simulink model "EKF_MODEL_needfix"  (R2023b)
settings: Solver=ode23tb  StartTime=0.0  StopTime=30  FixedStep=.001  RelTol=2e-1  EnableMultiTasking=on
StartFcn:
  | %tic
StopFcn:
  | %toc
model workspace (MAT data in the model file):
  DLCXref = [0 6.1 6.2 18 33 33.5 45 50 60]
  DLCXrefStanley = [0 1.2 2.4 3.6 4.8 6 7.2 8.4 9.44987166868 10.0991210544 10.1 10.1008789456 ... (38 elements, 1x38)]
  DLCYref = [0 0 -5 -3.875 -3.5 1 0 0 0]
  DLCYrefStanley = [0.1375 0.1375 0.1375 0.1375 0.1375 0.1375 0.1375 0.1375 -0.203439148031 -1.09615705337 -2.2 -3.30384294663 ... (38 elements, 1x38)]
  Downshift_Speeds = [9.5625 12.9375 16.3125 19.6875 23.0625 26.4375 29.8125 33.1875 36.5625 39.9375 43.3125 46.6875 ... (28 elements, 4x7)]
  EngRevLim = 7000
  Pedal_Positions = [0.1 0.4 0.5 0.9]
  Ts = 0.01
  Upshift_Speeds = [12.9375 16.3125 19.6875 33 26.4375 29.8125 33.1875 52.5 39.9375 43.3125 46.6875 77.25 ... (28 elements, 4x7)]
  VEH : object (value not decoded)
  a = 1.515
  b = 1.504
  for_ekf : mamfis (value not decoded)
  rayDirections = [0 0 0 0 0 0 0 0 0 0 0 0 ... (363 elements, 121x3)]
  rayLengths = [20 20 20 20 20 20 20 20 20 20 20 20 ... (121 elements, 121x1)]
  rayOrigins = [0.5 0.4 0.3 0.2 0.1 0 -0.1 -0.2 -0.3 -0.4 -0.5 0.5 ... (363 elements, 121x3)]
  theta = 1
  wf = 0.75
  wr = 1.25
symbols that are objects in the model workspace (value not decoded): VEH
undefined symbols (not defined in the file): DiscIntNeverNeededParam
libraries: simulink x14, autolibutils x7, slpidlib x2, vehdynlibdriver x2, vehdynlibviscommon x2, sim3dgroundtruthsensorlib x2, autolibtranscontrolscommon x1, autolibshared x1, sharedtransform x1, sharedTrackingLibrary x1, vehdynlibscenariocommon x1, vehdynlibsens x1
(part 3 of 4)

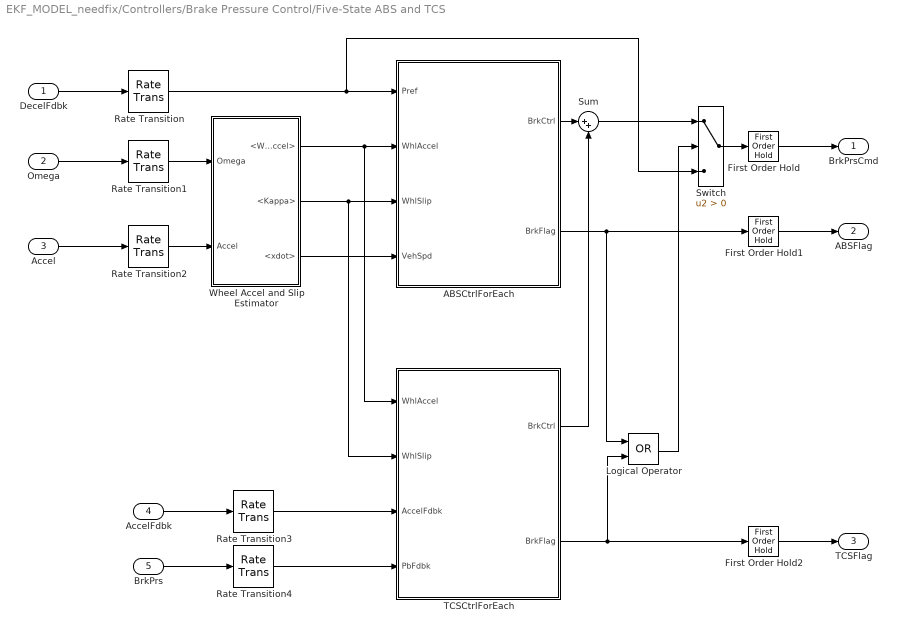
== system EKF_MODEL_needfix/Controllers/Brake Pressure Control/Five-State ABS and TCS ==
  DecelFdbk : Inport
  Omega : Inport  Port=2
  Accel : Inport  Port=3
  AccelFdbk : Inport  Port=4
  BrkPrs : Inport  Port=5
  ABSCtrlForEach : Subsystem  mask(Five-State ABS Control){Re=0.323, KappaOpt=-0.12, WhlAccelOpt=[-9.8,-9.8,-20,-20], v1=0, v5=0.55, v4=1, a2=-1.5, b=-1.5, A=4.5, a1=3.6, aMode=2}
      mask prompts: Re "Wheel effective radius, Re [m]:"; KappaOpt "Desired wheel slip ratio, KappaOpt [-]:"; WhlAccelOpt "Desired wheel acceleration, WhlAccelOpt [m/s^2]:"; v1 "Braking realease command, v1 [-]:"; v5 "Braking hold command, v5 [-]:"; v4 "Braking add command, v4 [-]:"; a2 "Threshold of State 1, a2 [m/s^2]:"; b "Threshold of State 2, b [m/s^2]:"; A "Threshold of State 3 and 4, A [m/s^2]:"; a1 "Threshold of State 5, a1 [m/s^2]:"
      mask help: This block determines brake pressure varying rate for each wheel once the ABS controller is activated. During ABS control, only wheel speed is directly regulated.
      mask init:
      | [~]=vehdynicon('vehdynblk',gcb);
      mask DialogControl vehParamGroup Prompt: Vehicle Parameter
      mask DialogControl ParameterGroupVar Prompt: Desired Control Parameters
      mask DialogControl Container3 Prompt: Braking Pressure Rates
      mask DialogControl Container4 Prompt: Wheel Acceleration Thresholds
  First Order Hold : FirstOrderHold  ErrorTolerance=.01
  First Order Hold1 : FirstOrderHold  ErrorTolerance=1
  First Order Hold2 : FirstOrderHold  ErrorTolerance=1
  Logical Operator : Logic  Operator=OR  AllPortsSameDT=off  OutDataTypeStr=boolean
  Rate Transition{,1..4} (5 alike) : RateTransition  OutPortSampleTime=.001
  Sum : Sum  Inputs=|++
  Switch : Switch  Criteria=u2 > Threshold  SaturateOnIntegerOverflow=off  InputSameDT=off
  TCSCtrlForEach : Subsystem  mask(Five-State TCS Control){Re=0.323, KappaOpt=0.12, WhlAccelOpt=[11, 11, 11, 11], v1=1.5, v5=-0.5, v4=-1.2, a2=-6, b=-10, A=-11, a1=-9, aMode=2}
      mask prompts: Re "Wheel effective radius, Re [m]:"; KappaOpt "Desired wheel slip ratio, KappaOpt [-]:"; WhlAccelOpt "Desired wheel acceleration, WhlAccelOpt [m/s^2]:"; v1 "Braking pressure rising rate, v1 [-]:"; v5 "Secondary braking pressure declining rate, v5 [-]:"; v4 "Braking pressure declining rate, v4 [-]:"; a2 "Threshold of State 1, a2 [m/s^2]:"; b "Threshold of State 2, b [m/s^2]:"; A "Threshold of State 3 and 4, A [m/s^2]:"; a1 "Threshold of State 5, a1 [m/s^2]:"
      mask help: This block determines brake pressure varying rate for each wheel once the TCS controller is activated. During TCS control, only wheel speed is directly regulated.
      mask init:
      | [~]=vehdynicon('vehdynblk',gcb);
      mask DialogControl vehParamGroup Prompt: Vehicle Parameter
      mask DialogControl ParameterGroupVar Prompt: Desired Control Parameters
      mask DialogControl Container3 Prompt: Braking Pressure Rates
      mask DialogControl Container4 Prompt: Wheel Acceleration Thresholds
  Wheel Accel and Slip Estimator : Subsystem
  BrkPrsCmd : Outport
  ABSFlag : Outport  Port=2  PortDimensions=4
  TCSFlag : Outport  Port=3  PortDimensions=4
  wires:
  Omega/1 -> Rate Transition1/1
  Accel/1 -> Rate Transition2/1
  DecelFdbk/1 -> Rate Transition/1
  Wheel Accel and Slip Estimator/1(<WhlAccel>) -> TCSCtrlForEach/1(WhlAccel), ABSCtrlForEach/2(WhlAccel)
  Wheel Accel and Slip Estimator/2(<Kappa>) -> TCSCtrlForEach/2(WhlSlip), ABSCtrlForEach/3(WhlSlip)
  Wheel Accel and Slip Estimator/3(<xdot>) -> ABSCtrlForEach/4(VehSpd)
  ABSCtrlForEach/2(BrkFlag) -> First Order Hold1/1, Logical Operator/1
  First Order Hold/1 -> BrkPrsCmd/1
  Rate Transition/1 -> Switch/3, ABSCtrlForEach/1(Pref)
  Rate Transition1/1 -> Wheel Accel and Slip Estimator/1(Omega)
  Rate Transition2/1 -> Wheel Accel and Slip Estimator/2(Accel)
  First Order Hold1/1 -> ABSFlag/1
  Switch/1 -> First Order Hold/1
  AccelFdbk/1 -> Rate Transition3/1
  First Order Hold2/1 -> TCSFlag/1
  TCSCtrlForEach/2(BrkFlag) -> First Order Hold2/1, Logical Operator/2
  Rate Transition3/1 -> TCSCtrlForEach/3(AccelFdbk)
  TCSCtrlForEach/1(BrkCtrl) -> Sum/2
  ABSCtrlForEach/1(BrkCtrl) -> Sum/1
  BrkPrs/1 -> Rate Transition4/1
  Rate Transition4/1 -> TCSCtrlForEach/4(PbFdbk)
  Sum/1 -> Switch/1
  Logical Operator/1 -> Switch/2

== system EKF_MODEL_needfix/Controllers/Brake Pressure Control/Open Loop ==
  DecelFdbk : Inport
  Constant : Constant  Value=false
  Selector : Selector  InputPortWidth=1  IndexOptions=Index vector (dialog)  Indices=[1 1 1 1]  OutputSizes=1
  Selector1 : Selector  InputPortWidth=1  IndexOptions=Index vector (dialog)  Indices=[1 1 1 1]  OutputSizes=1
  BrkPrsCmd : Outport  VectorParamsAs1DForOutWhenUnconnected=off
  ABSFlag : Outport  Port=2
  wires:
  DecelFdbk/1 -> Selector1/1
  Selector1/1 -> BrkPrsCmd/1
  Constant/1 -> Selector/1
  Selector/1 -> ABSFlag/1

== system EKF_MODEL_needfix/Controllers/ECU/Torque Cmd ==
  DiffTrqCmd : Inport
  <Accel> : Inport  Port=2
  EngSpd : Inport  Port=3
  ABSFlag : Inport  Port=4
  Acc to Torque Request : Gain  Gain=150
  Constant : Constant  Value=0
  Max : MinMax  Function=max  Inputs=2
  OR : Logic  Operator=OR  Inputs=1  AllPortsSameDT=off  OutDataTypeStr=boolean
  Rev Limiter Control : Subsystem
  Signal Specification : SignalSpecification  Unit=rpm
  Switch : Switch  Criteria=u2 > Threshold  ZeroCross=off  SaturateOnIntegerOverflow=off  InputSameDT=off
  Unit Conversion : UnitConversion
  EngTrqCmd : Outport
  wires:
  Signal Specification/1 -> Rev Limiter Control/2(EngSpd)  "EngSpd"
  Unit Conversion/1 -> Signal Specification/1
  EngSpd/1 -> Unit Conversion/1
  <Accel>/1 -> Acc to Torque Request/1
  Acc to Torque Request/1 -> Rev Limiter Control/1(TrqCmd)
  DiffTrqCmd/1 -> Max/1
  Rev Limiter Control/1(TrqCmdRevLimited) -> Max/2
  Switch/1 -> EngTrqCmd/1
  Max/1 -> Switch/3
  ABSFlag/1 -> OR/1
  Constant/1 -> Switch/1
  OR/1 -> Switch/2

== system EKF_MODEL_needfix/Controllers/Transmission Controller/Driver - No Clutch ==
  GearReq : Inport
  Gear : Outport  VectorParamsAs1DForOutWhenUnconnected=off
  wires:
  GearReq/1 -> Gear/1

== system EKF_MODEL_needfix/Controllers/Transmission Controller/PRNDL Controller ==
  Accel : Inport
  BrkCmd : Inport  Port=2
  Omega : Inport  Port=3  Unit=rad/s
  EngSpd : Inport  Port=4  Unit=rad/s
  GearReq : Inport  Port=5
  ABSFlag : Inport  Port=6
  Cont LPF : autolibutils/Cont LPF  wc=4*2*pi  AbsoluteTolerance=auto  aMode=2
  Cont LPF1 : autolibutils/Cont LPF  wc=4*2*pi  AbsoluteTolerance=auto  aMode=2
  Gain : Gain  Gain=.3065/4
  OR : Logic  Operator=OR  Inputs=1  AllPortsSameDT=off  OutDataTypeStr=boolean
  Signal Specification1 : SignalSpecification  Unit=m/s
  Sum of Elements : Sum  Inputs=+
  Transmission Controller PRNDL : autolibtranscontrolscommon/Transmission Controller PRNDL  DriveMode=off  GearInit=1  LugSpd=1200  MinUpSpd=2000  tClutchUp=0.5  tClutchDn=0.5  tPark=120  VelUnit=km/hr  UpShSpd="reshape([20    25    30    45    35    45    40    55    40    55    55    65    50    60    65    75    60    65    80    90    70    75   120   150    85    85   150   185  20    25    30    45    35    45    40    55    40    55    55    65    50    60    65    75    60    65    80    90    70    75   120   150    85    85   150   185],4,7,2)"  UpLdBpt=[.1 .4 .75 1]  UpShBpt=1:7  UpPtBpt=[1 2]  DnShfSpd=reshape([9.5625 12.9375 16.3125 19.6875 23.0625 26.4375 29.8125 33.1875 36.5625 39.9375 43.3125 46.687499999999986 47.8125 51.187499999999986 54.562499999999986 57.9375 59.0625 62.4375 65.8125 69.1875 68.90625 72.84375 76.78125 80.71875 78.75 83.25 87.75 92.25 31.619930749150555 36.119930749150555 37.619930749150555 43.619930749150555 44.318578948924035 48.818578948924035 50.318578948924035 56.318578948924035 53.598360325681568 58.098360325681568 59.598360325681568 65.598360325681568 66.252607657623685 70.752607657623685 72.252607657623685 78.252607657623685 84.53096491487338 89.03096491487338 90.53096491487338 96.53096491487338 134.79644737231007 139.29644737231007 140.79644737231007 146.79644737231007 210.1946710584651 214.6946710584651 216.1946710584651 222.1946710584651],4,7,2)  DnShSpd=[10 15 25 30 40 55 75; 10 18 25 35 50 65 80; 12 18 21 55 65 75 85; 15 20 25 55 70 80 95]  DnLdBpt=[.1 .4 .75 1]  DnShBpt=2:8  DnPtBpt=[1 2]  POFS=zeros(4,1)  GOFS=zeros(1,7)  Ngears=8  aMode=2
  Gear : Outport  VectorParamsAs1DForOutWhenUnconnected=off
  wires:
  Gain/1 -> Cont LPF1/1
  Omega/1 -> Sum of Elements/1
  Sum of Elements/1 -> Gain/1
  ABSFlag/1 -> OR/1
  OR/1 -> Transmission Controller PRNDL/6
  Transmission Controller PRNDL/1 -> Gear/1
  GearReq/1 -> Transmission Controller PRNDL/1  "PRNDL"
  Accel/1 -> Transmission Controller PRNDL/2
  BrkCmd/1 -> Transmission Controller PRNDL/3
  Signal Specification1/1 -> Transmission Controller PRNDL/4
  EngSpd/1 -> Cont LPF/1
  Cont LPF1/1 -> Signal Specification1/1
  Cont LPF/1 -> Transmission Controller PRNDL/5

== system EKF_MODEL_needfix/Controllers/Transmission Controller/Paddles ==
  Accel : Inport
  EngSpd : Inport  Port=2  Unit=rad/s
  Add1 : Sum  Inputs=+-+
  Current Gear : UnitDelay  SampleTime=-1  HasFrameUpgradeWarning=on
  Data Type Conversion2 : DataTypeConversion  OutDataTypeStr=double  SaturateOnIntegerOverflow=off  RndMeth=Floor
  Debounce : autolibutils/Debounce  DbcOn_Cnts=10  DbcOff_Cnts=10  aMode=aMode
  Debounce1 : autolibutils/Debounce  DbcOn_Cnts=10  DbcOff_Cnts=10  aMode=aMode
  Demux : Demux  Outputs=2
  Detect Increase2 : simulink/Logic and Bit Operations/Detect Increase  vinit=0.0  OutDataTypeStr=boolean
  Logical Operator1 : Logic  Operator=XOR  Inputs=1  AllPortsSameDT=off  OutDataTypeStr=boolean
  Mux : Mux  Inputs=2
  Switch2 : Switch  Criteria=u2 > Threshold  SaturateOnIntegerOverflow=off  InputSameDT=off
  Gear : Outport  VectorParamsAs1DForOutWhenUnconnected=off
  wires:
  Debounce/1 -> Mux/1
  Mux/1 -> Detect Increase2/1
  Logical Operator1/1 -> Switch2/2
  Data Type Conversion2/1 -> Demux/1
  Demux/1 -> Add1/1
  Demux/2 -> Add1/2
  Current Gear/1 -> Add1/3, Switch2/3
  Switch2/1 -> Gear/1, Current Gear/1
  Debounce1/1 -> Mux/2
  Add1/1 -> Switch2/1
  Detect Increase2/1 -> Data Type Conversion2/1, Logical Operator1/1
  EngSpd/1 -> Debounce1/1
  Accel/1 -> Debounce/1

== system EKF_MODEL_needfix/Controllers/Transmission Controller/Transmission Controller ==
  Accel : Inport
  EngSpd : Inport  Port=2  Unit=rad/s
  Omega : Inport  Port=3  Unit=rad/s
  10ms Function-Call Generator : simulink/Ports & Subsystems/Function-Call Generator  sample_time=0.01  numberOfIterations=1  DisallowWideOutput=off
  Data Type Conversion : DataTypeConversion  SaturateOnIntegerOverflow=off  RndMeth=Floor
  First Order Hold : FirstOrderHold  ErrorTolerance=.1
  Rate Transition : RateTransition  Deterministic=off
  Rate Transition1 : RateTransition  Deterministic=off
  Rate Transition2 : RateTransition  Deterministic=off
  Signal Specification : SignalSpecification  Unit=rpm
  TCM : Subsystem
  Unit Conversion : UnitConversion
  Gear : Outport  VectorParamsAs1DForOutWhenUnconnected=off
  wires:
  TCM/1(GearCmd) -> Data Type Conversion/1
  Rate Transition/1 -> TCM/1(AccCmd)
  10ms Function-Call Generator/1 -> TCM/Trigger
  Accel/1 -> Rate Transition/1
  Omega/1 -> Rate Transition2/1
  Rate Transition1/1 -> TCM/2(EngSpd)
  First Order Hold/1 -> Gear/1
  Unit Conversion/1 -> Signal Specification/1
  Signal Specification/1 -> Rate Transition1/1  "EngSpd"
  EngSpd/1 -> Unit Conversion/1
  Data Type Conversion/1 -> First Order Hold/1
  Rate Transition2/1 -> TCM/3(Omega)

== system EKF_MODEL_needfix/Driver Commands/Driver Commands/Longitudinal Driver ==
  VehRef : Inport
  VehFdbk : Inport  Port=2
  Bus Creator2 : BusCreator  Inputs=5
  Bus Selector2 : BusSelector  OutputSignals=Body.BdyFrm.Cg.Vel.xdot,Body.InertFrm.Cg.Disp.X
  Bus Selector3 : BusSelector  OutputSignals=SteerOvrCmd,LngRef,LtrlRef
  Dead Zone1 : DeadZone  LowerValue=-.1  UpperValue=.1
  Ground1 : Ground
  Ground2 : Ground
  Longitudinal Driver : autolibshared/Longitudinal Driver  extAccelOvr=off  extDecelOvr=off  extAccelHld=off  extDecelHld=off  extAccelZero=off  extDecelZero=off  cntrlType=Predictive  shftType=Reverse, Neutral, Drive  velUnits=m/s  gearOut=on  Kp=5  Ki=5  Kff=.1  Kg=0  VehVelVec=[0 100]  KffVec=[.1 .1]  KpVec=[10 10]  KiVec=[5 5]  KgVec=[0 0]  m=VEH.Mass  Kpt=3000  tau=.5  L=2  aR=200  bR=2.5  cR=.5  g=9.81  vnom=5  Kaw=1  tauerr=.1  tauPt=2  GearInit=0  tShift=.1  pdlVec=[0.1 0.4 0.5 0.9]  upShftTbl=[-1 12.9375 26.4375 39.9375 51.18749999999999 62.4375 72.84375 83.25;-1 16.3125 29.8125 43.3125 54.5624 65.8125 76.78125 87.75;-1 19.6875 33.1875 46.68749999999999 57.9375 69.1875 80.71875 92.25;-1 33 52.5 77.25 100.5 138.75 161.875 185]  dwnShftTbl=[1 9.5625 23.0625 36.5625 47.8125 59.0625 68.90625 78.75;1 12.9375 26.4375 39.9375 51.18749999999999 62.4375 72.84375 83.25;1 16.3125 29.8125 43.3125 54.562499 65.8125 76.78125 87.75;1 19.6875 33.1875 46.68749999999999 57.9375 69.1875 80.71875 92.25]  tClutch=.5  tRev=.5  tPark=120  aMode=2  UpGearVec="[0  1  2  3  4  5  6  7]"  DownGearVec="[1  2  3  4  5  6  7  8]"
      settings: LibrarySourceBlock=vehdynlibdriver/Longitudinal Driver
  Mux : Mux  Inputs=3
  Signal Copy : SignalConversion  OverrideOpt=off
  Terminator1 : Terminator
  Unit Conversion : UnitConversion
  Driver : Outport  VectorParamsAs1DForOutWhenUnconnected=off
  wires:
  VehRef/1 -> Bus Selector3/1
  Signal Copy/1 -> Bus Creator2/1  "SteerCmd"
  Longitudinal Driver/2 -> Bus Creator2/2  "AccelCmd"
  Dead Zone1/1 -> Longitudinal Driver/2
  Bus Selector3/2 -> Unit Conversion/1  "<LngRef>"
  Ground1/1 -> Longitudinal Driver/3
  Bus Selector2/1 -> Dead Zone1/1  "<xdot>"
  Bus Creator2/1 -> Driver/1
  Longitudinal Driver/1 -> Terminator1/1
  Longitudinal Driver/3 -> Bus Creator2/3  "DecelCmd"
  VehFdbk/1 -> Bus Selector2/1
  Bus Selector3/1 -> Signal Copy/1  "<SteerOvrCmd>"
  Ground2/1 -> Mux/3
  Bus Selector2/2 -> Mux/1  "<X>"
  Mux/1 -> Bus Creator2/5  "Ref"
  Bus Selector3/3 -> Mux/2  "<LtrlRef>"
  Longitudinal Driver/4 -> Bus Creator2/4  "GearCmd"
  Unit Conversion/1 -> Longitudinal Driver/1

== system EKF_MODEL_needfix/Driver Commands/Driver Commands/Open Loop ==
  VehFdbk : Inport
  SteerCmd : Inport  Port=2
  Accel : Inport  Port=3  Unit=one
  Brake : Inport  Port=4  Unit=1
  Gear : Inport  Port=5  Unit=1
  Bus Creator1 : BusCreator  Inputs=4
  Signal Specification : SignalSpecification  Unit=rad
  Signal Specification1 : SignalSpecification  Unit=1
  Signal Specification2 : SignalSpecification  Unit=1
  Signal Specification3 : SignalSpecification  Unit=1
  Terminator : Terminator
  Unit Conversion{,1..3} (4 alike) : UnitConversion
  Driver : Outport  VectorParamsAs1DForOutWhenUnconnected=off
  wires:
  Unit Conversion3/1 -> Signal Specification3/1
  Unit Conversion2/1 -> Signal Specification2/1
  Unit Conversion/1 -> Signal Specification/1
  Bus Creator1/1 -> Driver/1
  Accel/1 -> Unit Conversion1/1
  VehFdbk/1 -> Terminator/1
  SteerCmd/1 -> Unit Conversion/1
  Unit Conversion1/1 -> Signal Specification1/1
  Brake/1 -> Unit Conversion2/1
  Gear/1 -> Unit Conversion3/1
  Signal Specification/1 -> Bus Creator1/1  "SteerCmd"
  Signal Specification1/1 -> Bus Creator1/2  "AccelCmd"
  Signal Specification2/1 -> Bus Creator1/3  "DecelCmd"
  Signal Specification3/1 -> Bus Creator1/4  "GearCmd"

== system EKF_MODEL_needfix/Driver Commands/Driver Commands/Predictive Driver ==
  VehRef : Inport
  VehFdbk : Inport  Port=2
  Bus Creator1 : BusCreator  Inputs=5
  Bus Selector : BusSelector  OutputSignals=Body.BdyFrm.Cg.Vel.xdot,Body.InertFrm.Cg.Disp.Y,Body.BdyFrm.Cg.Vel.ydot,Body.InertFrm.Cg.Ang.psi,Body.BdyFrm.Cg.AngVel.r,Body.InertFrm.Cg.Disp.X
  Bus Selector1 : BusSelector  OutputSignals=LngRef,LtrlRef,EnblSteerCmd,SteerOvrCmd,AccelZero
  Dead Zone : DeadZone  LowerValue=-.5  UpperValue=.5  ZeroCross=off
  Grade : Constant  Value=0  SampleTime=-1
  Linear Predictive Driver : vehdynlibdriver/Predictive Driver  extAccelOvr=off  extDecelOvr=off  extAccelHld=off  extDecelHld=off  extAccelZero=on  extDecelZero=off  extSteerOvr=on  extSteerHld=off  extSteerZero=off  cntrlType=Predictive  cntrlTypeLat=Predictive  shftType=Reverse, Neutral, Drive  coordMode=SAE J670 (Z-down)  refType=Reference pose  velUnits=m/s  angUnits=rad  gearOut=on  steerOut=on  Kp=3  Ki=1  Kff=1  Kg=0  VehVelVec=[0 100]  KffVec=[.1 .1]  KpVec=[10 10]  KiVec=[5 5]  KgVec=[0 0]  vnom=5  Kaw=1  tauerr=.075  tau=.15  L=6  Kpt=20000  aR=200  bR=2.5  cR=.5  g=9.81  vecPose=off  dynamMode=on  PositionGainF=2.5  PositionGainR=2.5  YawRateGain=.2  DelayGain=.2  enableDrift=off  BetaRef=20*pi/180  KpBeta=1  KpDrift=2  KdDrift=1  KpPsi=6  KOmega=30  tOmega=1  a=VEH.FrontAxlePositionfromCG  b=VEH.RearAxlePositionfromCG  m=VEH.Mass  Cy_f=5000  Cy_r=7000  I=VEH.YawMomentInertia  Ksteer=18  theta=60*pi/180  Idl=1  Re=.3  lambda_mu=1  GearInit=0  tShift=.1  pdlVec=[0.1 0.4 0.5 0.9]  upShftTbl=[-1 12.9375 26.4375 39.9375 51.18749999999999 62.4375 72.84375 83.25;-1 16.3125 29.8125 43.3125 54.5624 65.8125 76.78125 87.75;-1 19.6875 33.1875 46.68749999999999 57.9375 69.1875 80.71875 92.25;-1 33 52.5 77.25 100.5 138.75 161.875 185]  dwnShftTbl=[-1 12.9375 26.4375 39.9375 51.18749999999999 62.4375 72.84375 83.25;-1 16.3125 29.8125 43.3125 54.5624 65.8125 76.78125 87.75;-1 19.6875 33.1875 46.68749999999999 57.9375 69.1875 80.71875 92.25;-1 33 52.5 77.25 100.5 138.75 161.875 185]  tClutch=.5  tRev=.5  tPark=120  UpGearVec="[0  1  2  3  4  5  6  7]"  DownGearVec="[1  2  3  4  5  6  7  8]"  aMode=2
  Mux : Mux  Inputs=3
  Terminator : Terminator
  Unit Conversion : UnitConversion
  Z : Constant  Value=0  SampleTime=-1
  Driver : Outport  VectorParamsAs1DForOutWhenUnconnected=off
  wires:
  Mux/1 -> Bus Creator1/5  "Ref"
  Bus Selector/6 -> Mux/1  "<X>"
  Linear Predictive Driver/5 -> Bus Creator1/4  "GearCmd"
  Bus Selector/3 -> Linear Predictive Driver/9  "<ydot>"
  Linear Predictive Driver/1 -> Terminator/1
  Bus Selector/5 -> Linear Predictive Driver/11  "<r>"
  Bus Selector1/2 -> Mux/2, Linear Predictive Driver/2  "<LtrlRef>"
  Z/1 -> Mux/3
  Grade/1 -> Linear Predictive Driver/6
  Bus Selector/1 -> Dead Zone/1  "<xdot>"
  Bus Selector/4 -> Linear Predictive Driver/10  "<psi>"
  Linear Predictive Driver/4 -> Bus Creator1/3  "DecelCmd"
  Dead Zone/1 -> Linear Predictive Driver/7
  VehFdbk/1 -> Bus Selector/1
  VehRef/1 -> Bus Selector1/1  "xdotref"
  Linear Predictive Driver/2 -> Bus Creator1/1  "SteerCmd"
  Bus Creator1/1 -> Driver/1
  Linear Predictive Driver/3 -> Bus Creator1/2  "AccelCmd"
  Bus Selector/2 -> Linear Predictive Driver/8  "<Y>"
  Bus Selector1/1 -> Unit Conversion/1  "<LngRef>"
  Bus Selector1/5 -> Linear Predictive Driver/5  "<AccelZero>"
  Bus Selector1/3 -> Linear Predictive Driver/3  "<EnblSteerCmd>"
  Bus Selector1/4 -> Linear Predictive Driver/4  "<SteerOvrCmd>"
  Unit Conversion/1 -> Linear Predictive Driver/1

== system EKF_MODEL_needfix/Driver Commands/Driver Commands/Predictive Stanley Driver ==
  VehRef : Inport
  VehFdbk : Inport  Port=2
  Bus Creator1 : BusCreator  Inputs=6
  Bus Selector : BusSelector  OutputSignals=Body.BdyFrm.Cg.Vel.xdot,Body.InertFrm.Cg.Disp.X,Body.InertFrm.Cg.Disp.Y,Body.InertFrm.Cg.Ang.psi,Body.BdyFrm.Cg.AngVel.r
  Bus Selector1 : BusSelector  OutputSignals=LngRef,PoseRef,EnblSteerCmd,SteerOvrCmd,SteerHld,SteerZero,EnblAccelOvr,AccelOvrCmd,AccelHld,AccelZero,EnblDecelCmd,DecelOvrCmd,DecelHld,DecelZero,CurvRef
  Constant : Constant  Value=false  SampleTime=-1
  Dead Zone : DeadZone  LowerValue=-.5  UpperValue=.5  ZeroCross=off
  Grade : Constant  Value=0  SampleTime=-1
  Linear Predictive Driver : vehdynlibdriver/Predictive Driver  extAccelOvr=on  extDecelOvr=on  extAccelHld=on  extDecelHld=on  extAccelZero=on  extDecelZero=on  extSteerOvr=on  extSteerHld=on  extSteerZero=on  cntrlType=Predictive  cntrlTypeLat=Stanley  shftType=Reverse, Neutral, Drive  coordMode=SAE J670 (Z-down)  refType=Reference pose  velUnits=m/s  angUnits=rad  gearOut=on  steerOut=on  Kp=3  Ki=1  Kff=1  Kg=0  VehVelVec=[0 100]  KffVec=[.1 .1]  KpVec=[10 10]  KiVec=[5 5]  KgVec=[0 0]  vnom=5  Kaw=1  tauerr=.075  tau=.15  L=6  Kpt=20000  aR=200  bR=2.5  cR=.5  g=9.81  vecPose=on  dynamMode=on  PositionGainF=2  PositionGainR=2  YawRateGain=.2  DelayGain=.01  enableDrift=off  BetaRef=20*pi/180  KpBeta=1  KpDrift=2  KdDrift=1  KpPsi=6  KOmega=30  tOmega=1  a=VEH.FrontAxlePositionfromCG  b=VEH.RearAxlePositionfromCG  m=VEH.Mass  Cy_f=160000  Cy_r=7000  I=VEH.YawMomentInertia  Ksteer=18  theta=60*pi/180  Idl=1  Re=.3  lambda_mu=1  GearInit=0  tShift=.1  pdlVec=[0.1 0.4 0.5 0.9]  upShftTbl=[-1 12.9375 26.4375 39.9375 51.18749999999999 62.4375 72.84375 83.25;-1 16.3125 29.8125 43.3125 54.5624 65.8125 76.78125 87.75;-1 19.6875 33.1875 46.68749999999999 57.9375 69.1875 80.71875 92.25;-1 33 52.5 77.25 100.5 138.75 161.875 185]  dwnShftTbl=[-1 12.9375 26.4375 39.9375 51.18749999999999 62.4375 72.84375 83.25;-1 16.3125 29.8125 43.3125 54.5624 65.8125 76.78125 87.75;-1 19.6875 33.1875 46.68749999999999 57.9375 69.1875 80.71875 92.25;-1 33 52.5 77.25 100.5 138.75 161.875 185]  tClutch=.5  tRev=.5  tPark=120  UpGearVec="[0  1  2  3  4  5  6  7]"  DownGearVec="[1  2  3  4  5  6  7  8]"  aMode=2
  Memory : Memory  InitialCondition=[VEH.InitialLongPosition VEH.InitialLatPosition VEH.InitialYawAngle]  InheritSampleTime=on
  Memory1 : Memory  InheritSampleTime=on
  Memory2 : Memory  InheritSampleTime=on
  Mux : Mux  Inputs=3
  Mux1 : Mux  Inputs=3
  Terminator : Terminator
  Unit Conversion : UnitConversion
  Z : Constant  Value=0  SampleTime=-1
  Driver : Outport  VectorParamsAs1DForOutWhenUnconnected=off
  wires:
  Bus Selector1/11 -> Linear Predictive Driver/11  "<EnblDecelCmd>"
  Mux/1 -> Memory/1
  Linear Predictive Driver/3 -> Bus Creator1/2  "AccelCmd"
  Bus Selector/2 -> Mux1/1, Mux/1  "<X>"
  Bus Selector1/13 -> Linear Predictive Driver/13  "<DecelHld>"
  Bus Selector1/10 -> Linear Predictive Driver/10  "<AccelZero>"
  Linear Predictive Driver/5 -> Bus Creator1/4  "GearCmd"
  VehRef/1 -> Bus Selector1/1
  Bus Selector1/6 -> Linear Predictive Driver/6  "<SteerZero>"
  Bus Creator1/1 -> Driver/1
  Bus Selector1/4 -> Linear Predictive Driver/4  "<SteerOvrCmd>"
  Linear Predictive Driver/1 -> Terminator/1
  Bus Selector1/3 -> Linear Predictive Driver/3  "<EnblSteerCmd>"
  Constant/1 -> Bus Creator1/6  "IgnSwtch"
  Bus Selector1/1 -> Unit Conversion/1  "<LngRef>"
  Linear Predictive Driver/4 -> Bus Creator1/3  "DecelCmd"
  Bus Selector1/8 -> Linear Predictive Driver/8  "<AccelOvrCmd>"
  Bus Selector/3 -> Mux1/2, Mux/2  "<Y>"
  Bus Selector1/5 -> Linear Predictive Driver/5  "<SteerHld>"
  Linear Predictive Driver/2 -> Bus Creator1/1  "SteerCmd"
  Bus Selector1/7 -> Linear Predictive Driver/7  "<EnblAccelOvr>"
  Bus Selector/4 -> Mux/3  "<psi>"
  Bus Selector1/9 -> Linear Predictive Driver/9  "<AccelHld>"
  Bus Selector1/2 -> Linear Predictive Driver/2  "<PoseRef>"
  Bus Selector1/15 -> Linear Predictive Driver/16  "<CurvRef>"
  Bus Selector1/12 -> Linear Predictive Driver/12  "<DecelOvrCmd>"
  Grade/1 -> Linear Predictive Driver/15
  Bus Selector1/14 -> Linear Predictive Driver/14  "<DecelZero>"
  Unit Conversion/1 -> Linear Predictive Driver/1
  Bus Selector/1 -> Memory2/1  "<xdot>"
  Bus Selector/5 -> Memory1/1  "<r>"
  VehFdbk/1 -> Bus Selector/1
  Memory/1 -> Linear Predictive Driver/18
  Memory1/1 -> Linear Predictive Driver/19
  Memory2/1 -> Dead Zone/1
  Z/1 -> Mux1/3
  Mux1/1 -> Bus Creator1/5  "Ref"
  Dead Zone/1 -> Linear Predictive Driver/17

== system EKF_MODEL_needfix/Environment/Ground Feedback/3D Engine ==
  Friction : Inport
  VehFdbk : Inport  Port=2
  3D Engine Source : Subsystem  Variant=on  VariantControl=Choice  mask(Terrain Source){terrType=Single point}
      mask prompts: terrType "Terrain feedback type:"
      mask help:
      | This variant subsystem provides the option for:
      | - a single point of contact for each wheel with minimal post-processing ideal for smooth surfaces and maximum run-time performance.
      | - multiple points of contact per wheel which may be used when interested in non-smooth terrain at a higher computational cost.
      mask TypeOptions terrType: Single point | Multiple points
  Bus Creator2 : BusCreator  Inputs=4
  Bus Creator3 : BusCreator  Inputs=3
  Demux1 : Demux
  Signal Specification1 : SignalSpecification  Unit=1
  Ground : Outport  VectorParamsAs1DForOutWhenUnconnected=off
  wires:
  Signal Specification1/1 -> Demux1/1
  Demux1/1 -> Bus Creator2/1  "mu_FL"
  Demux1/3 -> Bus Creator2/3  "mu_RL"
  Demux1/4 -> Bus Creator2/4  "mu_RR"
  Demux1/2 -> Bus Creator2/2  "mu_FR"
  Bus Creator2/1 -> Bus Creator3/3  "mu"
  Bus Creator3/1 -> Ground/1
  Friction/1 -> Signal Specification1/1
  VehFdbk/1 -> 3D Engine Source/1(VehFdbk)
  3D Engine Source/1(z) -> Bus Creator3/1  "z"
  3D Engine Source/2(DCM) -> Bus Creator3/2  "DCM"

== system EKF_MODEL_needfix/Environment/Ground Feedback/Constant ==
  Friction : Inport
  Bus Creator : BusCreator  Inputs=4
  Bus Creator2 : BusCreator  Inputs=4
  Bus Creator3 : BusCreator  Inputs=3
  Constant1 : Constant  Value=zeros(4,1)
  Constant2 : Constant  Value=repmat(eye(3),1,1,4)  SampleTime=-1
  Demux : Demux
  Demux1 : Demux
  Signal Specification : SignalSpecification  Unit=m
  Signal Specification1 : SignalSpecification  Unit=1
  Ground : Outport  VectorParamsAs1DForOutWhenUnconnected=off
  wires:
  Constant1/1 -> Signal Specification/1
  Signal Specification/1 -> Demux/1
  Demux/4 -> Bus Creator/4  "G_RR_z"
  Demux/1 -> Bus Creator/1  "G_FL_z"
  Demux/3 -> Bus Creator/3  "G_RL_z"
  Demux/2 -> Bus Creator/2  "G_FR_z"
  Bus Creator/1 -> Bus Creator3/1  "z"
  Demux1/3 -> Bus Creator2/3  "mu_RL"
  Demux1/4 -> Bus Creator2/4  "mu_RR"
  Demux1/1 -> Bus Creator2/1  "mu_FL"
  Demux1/2 -> Bus Creator2/2  "mu_FR"
  Bus Creator2/1 -> Bus Creator3/3  "mu"
  Friction/1 -> Signal Specification1/1
  Signal Specification1/1 -> Demux1/1
  Bus Creator3/1 -> Ground/1
  Constant2/1 -> Bus Creator3/2  "DCM"

== system EKF_MODEL_needfix/Passenger Vehicle/Pedal Cluster and Cabin/Brake Pedal ==
  DecelCmd : Inport
  Constant1 : Constant  Value=-20
  Dead Zone1 : DeadZone  LowerValue=0  UpperValue=.01  ZeroCross=off
  Gain3 : Gain
  Integrator2 : Integrator  LimitOutput=on  UpperSaturationLimit=1  LowerSaturationLimit=0
  Switch1 : Switch  Criteria=u2 > Threshold  Threshold=.1  SaturateOnIntegerOverflow=off  InputSameDT=off
  DecelFdbk : Outport
  wires:
  Dead Zone1/1 -> Switch1/2, Gain3/1
  Constant1/1 -> Switch1/3
  Integrator2/1 -> DecelFdbk/1
  Gain3/1 -> Switch1/1
  Switch1/1 -> Integrator2/1
  DecelCmd/1 -> Dead Zone1/1

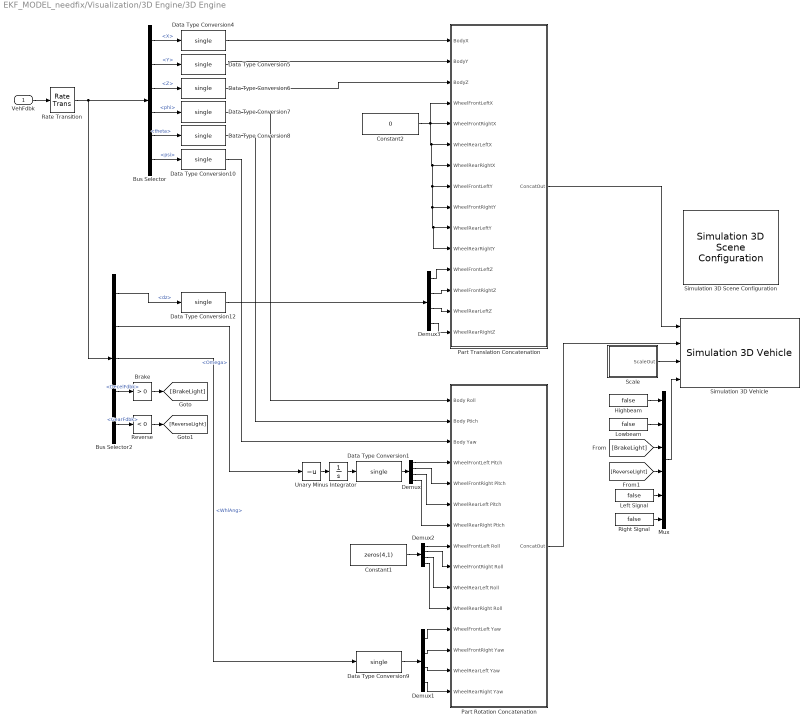
== system EKF_MODEL_needfix/Visualization/3D Engine/3D Engine ==
  VehFdbk : Inport
  Brake : simulink/Logic and Bit Operations/Compare To Constant  relop=>  const=0  OutDataTypeStr=boolean  ZeroCross=off
  Bus Selector : BusSelector  OutputSignals=Body.InertFrm.Geom.Disp.X,Body.InertFrm.Geom.Disp.Y,Body.InertFrm.Geom.Disp.Z,Body.InertFrm.Cg.Ang.phi,Body.InertFrm.Cg.Ang.theta,Body.InertFrm.Cg.Ang.psi
  Bus Selector2 : BusSelector  OutputSignals=Wheels.TireFrame.dz,Wheels.TireFrame.Omega,Driveline.WhlAng,Driver.DecelFdbk,Driver.GearFdbk
  Constant1 : Constant  Value=zeros(4,1)  OutDataTypeStr=single
  Constant2 : Constant  Value=0  OutDataTypeStr=single
  Data Type Conversion{1,4..10,12} (9 alike) : DataTypeConversion  OutDataTypeStr=single  SaturateOnIntegerOverflow=off  RndMeth=Floor
  Demux{,1..3} (4 alike) : Demux
  Highbeam : Constant  Value=false
  Integrator : Integrator  WrapState=on  WrappedStateUpperValue=2*pi  WrappedStateLowerValue=0  ZeroCross=off
  Left Signal : Constant  Value=false
  Lowbeam : Constant  Value=false
  Mux : Mux  Inputs=6
  Part Rotation Concatenation : Subsystem
  Part Translation Concatenation : Subsystem
  Rate Transition : RateTransition  OutPortSampleTime=dt3D
  Reverse : simulink/Logic and Bit Operations/Compare To Constant  relop=<  const=0  OutDataTypeStr=boolean  ZeroCross=off
  Right Signal : Constant  Value=false
  Scale : Subsystem
  Simulation 3D Scene Configuration : sim3dlib/Simulation 3D Scene Configuration  Priority=0  ProjectFormat=Default Scenes  SceneDesc=Double lane change  ProjectName=C:\Program Files\MATLAB\R2023b\toolbox\shared\sim3d_projects\automotive_project_windows\UE\WindowsNoEditor\VehicleSimulation.exe  ScenePath=/Game/Maps/HwStrght  UEProjPath=L:\Bsim3d\scm\automotive_project_UE4\2.23.0\src\main\AutoVrtlEnv\AutoVrtlEnv.uproject  EnableOpenDRIVE=off  vehTagList={'Scene Origin';'SimulinkVehicle1'}  vehTag=SimulinkVehicle1  FreeCameraInitialTranslation=[0, 0, 0]  FreeCameraDefaultInitialTranslation=[-6, 0, 2]  FreeCameraInitialRotation=[0, 0, 0]  FreeCameraDefaultInitialRotation=[0, -15, 0]  OpVisEn=off  Ts=dt3D  EnableWindow=on  EnableRemoteAccess=off  EnableWeather=off  SunAltitude=40.0  SunAzimuth=90  clouds=10  wind=1  fog=0  rain=0  EnableGeospatial=off  OriginHeight=200  OriginLatitude=40.744652  OriginLongitude=-73.988864  MapStyle=Aerial  AdditionalAssetIDs=[]  UseAdvancedSunSky=off  SolarTime=11  TimeZone=-5  Day=21  Month=9  Year=2022  UseDaylightSavingTime=on  DSTStartDay=10  DSTStartMonth=3  DSTEndDay=3  DSTEndMonth=11  DSTSwitchHour=2  sensorTag=MainCamera1  sensorId=1  sensorName=MainCamera1  mountLoc=Origin  offsetFlag=off  tmountOffset=[0, 0, 0]  rmountOffset=[0, 0, 0]  HorizontalResolution=1280  VerticalResolution=720  HorizontalFOV=60  mountPoint=[0 0 0]  mountOrientation=[0 0 0]  aMode=2  ID=1  GeoTrigger=Inactive
      settings: LibrarySourceBlock=vdynlib/Vehicle Scenarios/Sim3D/Sim3D Core/Simulation 3D Scene Configuration
  Simulation 3D Vehicle : sim3dautolib/Simulation 3D Vehicle  Priority=-1  PassVehMesh=Muscle car  MeshPath=/MathWorksSimulation/Vehicles/Muscle/Meshes/SK_MuscleCar.SK_MuscleCar  VehColor=Red  ActorName=SimulinkVehicle1  VehLightsControl=on  HeadlightColor=[ 1, 1, 1 ]  HighBeamIntensity=100000  LowBeamIntensity=60000  HighBeamConeAngle=1.22  LowBeamConeAngle=1.22  LeftHeadlightOrientation=[ 0, 0 ]  RightHeadlightOrientation=[ 0, 0 ]  BrakelightIntensity=500  ReverselightIntensity=500  SignallightIntensity=500  SignallightPeriod=1  SignalPulseWidth=50  Translation=[VEH.InitialLongPosition VEH.InitialLatPosition -VEH.InitialVertPosition; 0 0 0; 0 0 0; 0 0 0; 0 0 0]  Rotation=[VEH.InitialRollAngle VEH.InitialPitchAngle VEH.InitialYawAngle; 0 0 0; 0 0 0; 0 0 0; 0 0 0]  Scale=ones( 5, 3 )  SampleTime=dt3D  ActorType=SimulinkVehicle  ID=1  aMode=2  ActorTag=SimulinkVehicle1
  Unary Minus : UnaryMinus
  wires:
  Unary Minus/1 -> Integrator/1
  Bus Selector2/1 -> Data Type Conversion12/1  "<dz>"
  Rate Transition/1 -> Bus Selector/1, Bus Selector2/1
  Scale/1(ScaleOut) -> Simulation 3D Vehicle/3
  Demux/4 -> Part Rotation Concatenation/7(WheelRearRight Ptich)
  Demux/3 -> Part Rotation Concatenation/6(WheelRearLeft Pitch)
  Demux/2 -> Part Rotation Concatenation/5(WheelFrontRight Pitch)
  Demux/1 -> Part Rotation Concatenation/4(WheelFrontLeft Pitch)
  Constant1/1 -> Demux2/1
  Bus Selector/4 -> Data Type Conversion7/1  "<phi>"
  Part Rotation Concatenation/1(ConcatOut) -> Simulation 3D Vehicle/2
  Part Translation Concatenation/1(ConcatOut) -> Simulation 3D Vehicle/1
  Data Type Conversion12/1 -> Demux3/1
  Demux3/4 -> Part Translation Concatenation/15(WheelRearRightZ)
  Demux3/3 -> Part Translation Concatenation/14(WheelRearLeftZ)
  Demux3/1 -> Part Translation Concatenation/12(WheelFrontLeftZ)
  Demux3/2 -> Part Translation Concatenation/13(WheelFrontRightZ)
  VehFdbk/1 -> Rate Transition/1
  Data Type Conversion6/1 -> Part Translation Concatenation/3(BodyZ)
  Demux1/4 -> Part Rotation Concatenation/15(WheelRearRight Yaw)
  Demux1/3 -> Part Rotation Concatenation/14(WheelRearLeft Yaw)
  Demux2/1 -> Part Rotation Concatenation/8(WheelFrontLeft Roll)
  Demux2/2 -> Part Rotation Concatenation/9(WheelFrontRight Roll)
  Demux2/3 -> Part Rotation Concatenation/10(WheelRearLeft Roll)
  Demux2/4 -> Part Rotation Concatenation/11(WheelRearRight Roll)
  Bus Selector2/3 -> Data Type Conversion9/1  "<WhlAng>"
  Bus Selector2/2 -> Unary Minus/1  "<Omega>"
  Data Type Conversion9/1 -> Demux1/1
  Demux1/1 -> Part Rotation Concatenation/12(WheelFrontLeft Yaw)
  Demux1/2 -> Part Rotation Concatenation/13(WheelFrontRight Yaw)
  Integrator/1 -> Data Type Conversion1/1
  Data Type Conversion1/1 -> Demux/1
  Data Type Conversion8/1 -> Part Rotation Concatenation/2(Body Ptich)
  Data Type Conversion5/1 -> Part Translation Concatenation/2(BodyY)
  Data Type Conversion10/1 -> Part Rotation Concatenation/3(Body Yaw)
  Constant2/1 -> Part Translation Concatenation/5(WheelFrontRightX), Part Translation Concatenation/6(WheelRearLeftX), Part Translation Concatenation/7(WheelRearRightX), Part Translation Concatenation/8(WheelFrontLeftY), Part Translation Concatenation/9(WheelFrontRightY), Part Translation Concatenation/10(WheelRearLeftY), Part Translation Concatenation/11(WheelRearRightY), Part Translation Concatenation/4(WheelFrontLeftX)
  Data Type Conversion4/1 -> Part Translation Concatenation/1(BodyX)
  Data Type Conversion7/1 -> Part Rotation Concatenation/1(Body Roll)
  Bus Selector/1 -> Data Type Conversion4/1  "<X>"
  Bus Selector/2 -> Data Type Conversion5/1  "<Y>"
  Bus Selector/3 -> Data Type Conversion6/1  "<Z>"
  Bus Selector/6 -> Data Type Conversion10/1  "<psi>"
  Bus Selector/5 -> Data Type Conversion8/1  "<theta>"
  [BrakeLight] -> Mux/3
  Mux/1 -> Simulation 3D Vehicle/4
  Brake/1 -> [BrakeLight]
  Highbeam/1 -> Mux/1
  Reverse/1 -> [ReverseLight]
  [ReverseLight] -> Mux/4
  Lowbeam/1 -> Mux/2
  Right Signal/1 -> Mux/6
  Left Signal/1 -> Mux/5
  Bus Selector2/4 -> Brake/1  "<DecelFdbk>"
  Bus Selector2/5 -> Reverse/1  "<GearFdbk>"

== system EKF_MODEL_needfix/Visualization/3D Engine/3D Engine Disabled ==
  VehFdbk : Inport
  Terminator : Terminator
  wires:
  VehFdbk/1 -> Terminator/1

== system EKF_MODEL_needfix/Visualization/ISO 15037-1:2006/Disabled ==
  VehFdbk : Inport
  Terminator1 : Terminator
  wires:
  VehFdbk/1 -> Terminator1/1

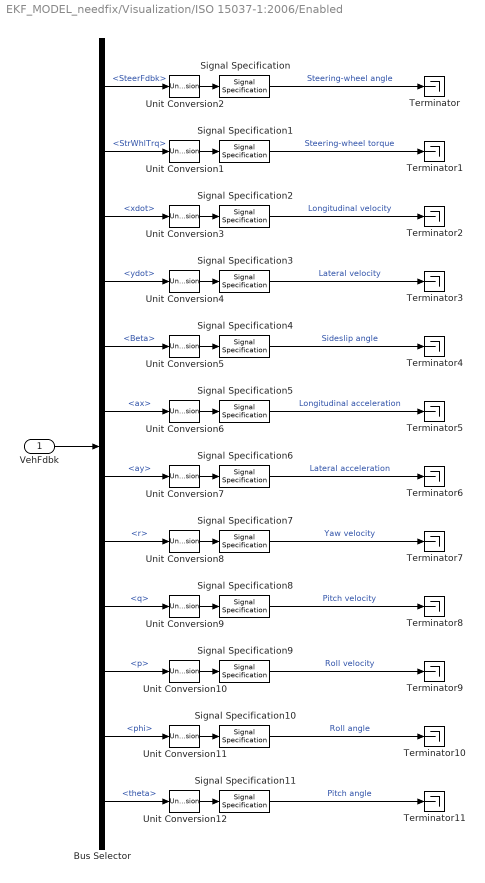
== system EKF_MODEL_needfix/Visualization/ISO 15037-1:2006/Enabled ==
  VehFdbk : Inport
  Bus Selector : BusSelector  OutputSignals=Driver.SteerFdbk,Steering.StrWhlTrq,Body.BdyFrm.Cg.Vel.xdot,Body.BdyFrm.Cg.Vel.ydot,Body.BdyFrm.Cg.Ang.Beta,Body.BdyFrm.Cg.Acc.ax,Body.BdyFrm.Cg.Acc.ay,Body.BdyFrm.Cg.AngVel.r,Body.BdyFrm.Cg.AngVel.q,Body.BdyFrm.Cg.AngVel.p,Body.InertFrm.Cg.Ang.phi,Body.InertFrm.Cg.Ang.theta
  Signal Specification{,4,10..11} (4 alike) : SignalSpecification  Unit=deg
  Signal Specification1 : SignalSpecification  Unit=N*m
  Signal Specification2 : SignalSpecification  Unit=km/h
  Signal Specification3 : SignalSpecification  Unit=m/s
  Signal Specification5 : SignalSpecification  Unit=m/s^2
  Signal Specification6 : SignalSpecification  Unit=m/s^2
  Signal Specification7 : SignalSpecification  Unit=deg/s
  Signal Specification8 : SignalSpecification  Unit=deg/s
  Signal Specification9 : SignalSpecification  Unit=deg/s
  Terminator{,1..11} (12 alike) : Terminator
  Unit Conversion{1..12} (12 alike) : UnitConversion
  wires:
  Bus Selector/12 -> Unit Conversion12/1  "<theta>"
  Signal Specification11/1 -> Terminator11/1  "Pitch angle"
  Unit Conversion12/1 -> Signal Specification11/1
  Bus Selector/11 -> Unit Conversion11/1  "<phi>"
  Unit Conversion11/1 -> Signal Specification10/1
  Signal Specification10/1 -> Terminator10/1  "Roll angle"
  Bus Selector/10 -> Unit Conversion10/1  "<p>"
  Signal Specification9/1 -> Terminator9/1  "Roll velocity"
  Unit Conversion10/1 -> Signal Specification9/1
  Bus Selector/9 -> Unit Conversion9/1  "<q>"
  Unit Conversion9/1 -> Signal Specification8/1
  Signal Specification8/1 -> Terminator8/1  "Pitch velocity"
  Bus Selector/8 -> Unit Conversion8/1  "<r>"
  Signal Specification7/1 -> Terminator7/1  "Yaw velocity"
  Unit Conversion8/1 -> Signal Specification7/1
  Bus Selector/7 -> Unit Conversion7/1  "<ay>"
  Unit Conversion7/1 -> Signal Specification6/1
  Signal Specification6/1 -> Terminator6/1  "Lateral acceleration"
  Bus Selector/6 -> Unit Conversion6/1  "<ax>"
  Signal Specification5/1 -> Terminator5/1  "Longitudinal acceleration"
  Unit Conversion6/1 -> Signal Specification5/1
  Bus Selector/5 -> Unit Conversion5/1  "<Beta>"
  Unit Conversion5/1 -> Signal Specification4/1
  Signal Specification4/1 -> Terminator4/1  "Sideslip angle"
  Bus Selector/4 -> Unit Conversion4/1  "<ydot>"
  Signal Specification3/1 -> Terminator3/1  "Lateral velocity"
  Unit Conversion4/1 -> Signal Specification3/1
  Bus Selector/3 -> Unit Conversion3/1  "<xdot>"
  Unit Conversion3/1 -> Signal Specification2/1
  Signal Specification2/1 -> Terminator2/1  "Longitudinal velocity"
  Signal Specification1/1 -> Terminator1/1  "Steering-wheel torque"
  Unit Conversion1/1 -> Signal Specification1/1
  Bus Selector/2 -> Unit Conversion1/1  "<StrWhlTrq>"
  Signal Specification/1 -> Terminator/1  "Steering-wheel angle"
  Unit Conversion2/1 -> Signal Specification/1
  VehFdbk/1 -> Bus Selector/1
  Bus Selector/1 -> Unit Conversion2/1  "<SteerFdbk>"

== system EKF_MODEL_needfix/model data/Subsystem/model data ==
  In1 : Inport
  In2 : Inport  Port=2
  Bus Selector : BusSelector  OutputSignals=xddot,yddot,r
  Bus Selector1 : BusSelector  OutputSignals=xdot,ydot,r
  Bus Selector2 : BusSelector  OutputSignals=SteerFdbk
  Bus Selector3 : BusSelector  OutputSignals=EngTrq
  Bus Selector4 : BusSelector  OutputSignals=Acc,pqr  OutputAsBus=on
  Mux : Mux  Inputs=3
  <imu> : Outport
  <body_a> : Outport  Port=2
  <SteerFdbk> : Outport  Port=3
  <EngTrq> : Outport  Port=4
  <xdot> : Outport  Port=5
  <ydot> : Outport  Port=6
  <r> : Outport  Port=7
  wires:
  Bus Selector2/1 -> <SteerFdbk>/1  "<SteerFdbk>"
  Bus Selector/2 -> Mux/2  "<yddot>"
  In1/1 -> Bus Selector3/1, Bus Selector2/1, Bus Selector1/1, Bus Selector/1
  Bus Selector1/3 -> <r>/1  "<r>"
  Bus Selector/1 -> Mux/1  "<xddot>"
  Bus Selector/3 -> Mux/3  "<r>"
  Bus Selector1/1 -> <xdot>/1  "<xdot>"
  Mux/1 -> <body_a>/1
  Bus Selector1/2 -> <ydot>/1  "<ydot>"
  In2/1 -> Bus Selector4/1
  Bus Selector4/1 -> <imu>/1
  Bus Selector3/1 -> <EngTrq>/1  "<EngTrq>"

== system EKF_MODEL_needfix/Controllers/Brake Pressure Control/Bang Bang ABS/Bang-bang controller ==
  in_1 : Inport
  Constant : Constant  Value=0
  Data Type Conversion1 : DataTypeConversion  OutDataTypeStr=double
  Data Type Conversion2 : DataTypeConversion  OutDataTypeStr=double
  Relational Operator : RelationalOperator  Operator=>  OutDataTypeStr=boolean
  Relational Operator1 : RelationalOperator  Operator=<  OutDataTypeStr=boolean
  Sum : Sum  Inputs=+-  InputSameDT=on  SaturateOnIntegerOverflow=on  OutDataTypeStr=Inherit: Same as first input
  out_1 : Outport  InitialOutput=0  VectorParamsAs1DForOutWhenUnconnected=off
  wires:
  Data Type Conversion2/1 -> Sum/2
  Data Type Conversion1/1 -> Sum/1
  Sum/1 -> out_1/1
  Relational Operator/1 -> Data Type Conversion1/1
  Relational Operator1/1 -> Data Type Conversion2/1
  Constant/1 -> Relational Operator/2, Relational Operator1/2
  in_1/1 -> Relational Operator1/1, Relational Operator/1

== system EKF_MODEL_needfix/Controllers/Brake Pressure Control/Bang Bang ABS/Kappa ==
  xdot : Inport
  Omega : Inport  Port=2  Partition=on  PartitionDimension=1  PartitionWidth=1  PartitionOffset=0
  For Each : ForEach  DisableCoverage=on
  MATLAB Function : MATLAB Function  TreatAsAtomicUnit=on
  KappaEst : Outport  ConcatenationDimension=1
  wires:
  MATLAB Function/1(KappaEst) -> KappaEst/1
  xdot/1 -> MATLAB Function/2(xdot)
  Omega/1 -> MATLAB Function/1(Omega)

== system EKF_MODEL_needfix/Controllers/Brake Pressure Control/Five-State ABS and TCS/ABSCtrlForEach ==
  Pref : Inport
  WhlAccel : Inport  Port=2
  WhlSlip : Inport  Port=3
  VehSpd : Inport  Port=4
  Constant7 : Constant  Value=WhlAccelOpt
  Constant8 : Constant  Value=KappaOpt
  For Each Subsystem : Subsystem  TreatAsAtomicUnit=on
  Gain : Gain  Gain=Re
  Saturation1 : Saturate  UpperLimit=1  LowerLimit=-1
  Selector : Selector  InputPortWidth=1  IndexOptions=Index vector (dialog)  Indices=[1 1 1 1]  OutputSizes=1
  Sum : Sum  Inputs=|+-
  Sum1 : Sum  Inputs=|+-
  BrkCtrl : Outport
  BrkFlag : Outport  Port=2
  wires:
  Gain/1 -> Sum/1
  Constant8/1 -> Sum1/2
  WhlSlip/1 -> Saturation1/1
  Constant7/1 -> Sum/2
  Sum1/1 -> For Each Subsystem/1(e1)
  WhlAccel/1 -> Gain/1
  Saturation1/1 -> Sum1/1
  For Each Subsystem/2(Flag) -> BrkFlag/1
  Pref/1 -> Selector/1
  VehSpd/1 -> For Each Subsystem/4(VehSpd)
  For Each Subsystem/1(Pb) -> BrkCtrl/1  "BrkPrsCmdCtrl"
  Selector/1 -> For Each Subsystem/3(Pref)
  Sum/1 -> For Each Subsystem/2(e2)

== system EKF_MODEL_needfix/Controllers/Brake Pressure Control/Five-State ABS and TCS/TCSCtrlForEach ==
  WhlAccel : Inport
  WhlSlip : Inport  Port=2
  AccelFdbk : Inport  Port=3
  PbFdbk : Inport  Port=4
  Constant7 : Constant  Value=WhlAccelOpt
  Constant8 : Constant  Value=KappaOpt
  For Each Subsystem : Subsystem  TreatAsAtomicUnit=on
  Gain : Gain  Gain=Re
  Interpreted MATLAB Function : MATLABFcn  MATLABFcn=abs((u(1)+u(2)) - (u(3) + u(4)))/2
  Saturation1 : Saturate  UpperLimit=1  LowerLimit=-1
  Selector : Selector  InputPortWidth=1  IndexOptions=Index vector (dialog)  Indices=[1 1 1 1]  OutputSizes=1
  Sum : Sum  Inputs=|+-
  Sum1 : Sum  Inputs=|+-
  BrkCtrl : Outport
  BrkFlag : Outport  Port=2
  wires:
  Gain/1 -> Sum/1
  Constant8/1 -> Sum1/2
  WhlSlip/1 -> Saturation1/1
  Constant7/1 -> Sum/2
  Sum1/1 -> For Each Subsystem/1(e1)
  WhlAccel/1 -> Gain/1
  Saturation1/1 -> Interpreted MATLAB Function/1, Sum1/1
  For Each Subsystem/2(Flag) -> BrkFlag/1
  AccelFdbk/1 -> Selector/1
  For Each Subsystem/1(Pb) -> BrkCtrl/1  "BrkPrsCmdCtrl"
  Selector/1 -> For Each Subsystem/4(AccelFdbk)
  Sum/1 -> For Each Subsystem/3(e2)
  Interpreted MATLAB Function/1 -> For Each Subsystem/2(Enb)
  PbFdbk/1 -> For Each Subsystem/5(PbFdbk)

== system EKF_MODEL_needfix/Controllers/Brake Pressure Control/Five-State ABS and TCS/Wheel Accel and Slip Estimator ==
  Omega : Inport
  Accel : Inport  Port=2
  Demux : Demux  Outputs=3
  Discrete-Time Integrator : DiscreteIntegrator  IntegratorMethod=Integration: Trapezoidal  SampleTime=-1  ICPrevOutput=DiscIntNeverNeededParam  ICPrevScaledInput=DiscIntNeverNeededParam
  Kappa : Subsystem  TreatAsAtomicUnit=on
  Terminator : Terminator
  Terminator1 : Terminator
  Wheel Accel : Subsystem  TreatAsAtomicUnit=on
  <WhlAccel> : Outport
  <Kappa> : Outport  Port=2
  <xdot> : Outport  Port=3
  wires:
  Accel/1 -> Demux/1
  Discrete-Time Integrator/1 -> <xdot>/1, Kappa/1(xdot)
  Demux/1 -> Discrete-Time Integrator/1
  Demux/2 -> Terminator/1
  Demux/3 -> Terminator1/1
  Omega/1 -> Kappa/2(Omega), Wheel Accel/1(Omega)
  Wheel Accel/1(WhlAccel) -> <WhlAccel>/1
  Kappa/1(KappaEst) -> <Kappa>/1

== system EKF_MODEL_needfix/Controllers/ECU/Torque Cmd/Rev Limiter Control ==
  TrqCmd : Inport
  EngSpd : Inport  Port=2
  1-D Lookup Table : Lookup_n-D  NumberOfTableDimensions=1  BreakpointsForDimension1=[1 1.01]  Table=[1 0]  ExtrapMethod=Clip  InternalRulePriority=Speed  RndMeth=Simplest
  Constant : Constant  Value=EngRevLim
  Product : Product
  Product1 : Product  Inputs=*/
  TrqCmdRevLimited : Outport  VectorParamsAs1DForOutWhenUnconnected=off
  wires:
  EngSpd/1 -> Product1/1
  Product/1 -> TrqCmdRevLimited/1
  1-D Lookup Table/1 -> Product/2
  TrqCmd/1 -> Product/1
  Constant/1 -> Product1/2
  Product1/1 -> 1-D Lookup Table/1

== system EKF_MODEL_needfix/Controllers/Transmission Controller/Transmission Controller/TCM ==
  AccCmd : Inport
  EngSpd : Inport  Port=2
  Omega : Inport  Port=3  Unit=rad/s
  function : TriggerPort  TriggerType=function-call  VariantControl=Variant
  Gain : Gain  Gain=.3065/4
  Neutral Select : Subsystem
  Signal Specification1 : SignalSpecification  Unit=m/s
  Signal Specification2 : SignalSpecification  Unit=km/hr
  Speed LPF : DiscreteTransferFcn  Numerator=[0.000000000000000 0.009950166250832 ]  Denominator=[1.000000000000000 -0.990049833749168 ]  mask(DiscretizedDiscreteTransferFcn){}
      mask init:
      | %zoh
  Sum of Elements : Sum  Inputs=+
  TCM Shift Controller : Stateflow chart  TreatAsAtomicUnit=on
  Unit Conversion1 : UnitConversion
  GearCmd : Outport  VectorParamsAs1DForOutWhenUnconnected=off
  wires:
  Signal Specification2/1 -> Speed LPF/1
  TCM Shift Controller/1(GearCmd) -> GearCmd/1  "GearCmd"
  AccCmd/1 -> Neutral Select/1(AccCmd), TCM Shift Controller/2(pedal)  "AccCmd"
  Neutral Select/1(Neutral Select) -> TCM Shift Controller/3(Neutral)
  EngSpd/1 -> Neutral Select/2(EngSpd)
  Speed LPF/1 -> TCM Shift Controller/1(speed)
  Unit Conversion1/1 -> Signal Specification2/1
  Omega/1 -> Sum of Elements/1
  Gain/1 -> Signal Specification1/1
  Signal Specification1/1 -> Unit Conversion1/1
  Sum of Elements/1 -> Gain/1

== system EKF_MODEL_needfix/Environment/Ground Feedback/3D Engine/3D Engine Source ==
  VehFdbk : Inport
  Multiple Points : Subsystem  VariantControl=terrType==2
  Single Point : Subsystem  VariantControl=terrType ==1
  z : Outport
  DCM : Outport  Port=2

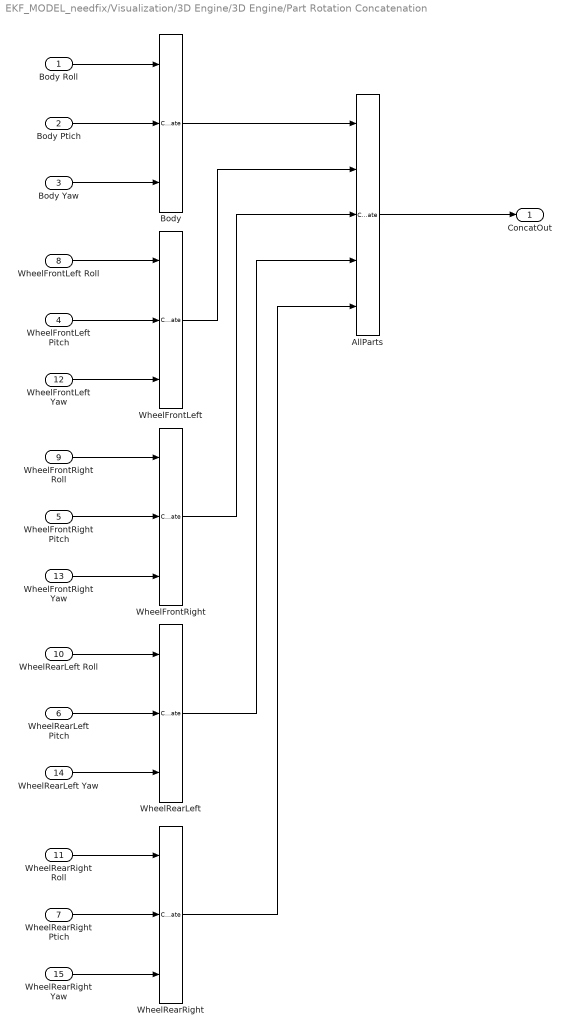
== system EKF_MODEL_needfix/Visualization/3D Engine/3D Engine/Part Rotation Concatenation ==
  Body Roll : Inport
  Body Ptich : Inport  Port=2
  Body Yaw : Inport  Port=3
  WheelFrontLeft Pitch : Inport  Port=4
  WheelFrontRight Pitch : Inport  Port=5
  WheelRearLeft Pitch : Inport  Port=6
  WheelRearRight Ptich : Inport  Port=7
  WheelFrontLeft Roll : Inport  Port=8
  WheelFrontRight Roll : Inport  Port=9
  WheelRearLeft Roll : Inport  Port=10
  WheelRearRight Roll : Inport  Port=11
  WheelFrontLeft Yaw : Inport  Port=12
  WheelFrontRight Yaw : Inport  Port=13
  WheelRearLeft Yaw : Inport  Port=14
  WheelRearRight Yaw : Inport  Port=15
  AllParts : Concatenate  NumInputs=5  Mode=Multidimensional array
  Body : Concatenate  NumInputs=3  Mode=Multidimensional array  ConcatenateDimension=2
  WheelFrontLeft : Concatenate  NumInputs=3  Mode=Multidimensional array  ConcatenateDimension=2
  WheelFrontRight : Concatenate  NumInputs=3  Mode=Multidimensional array  ConcatenateDimension=2
  WheelRearLeft : Concatenate  NumInputs=3  Mode=Multidimensional array  ConcatenateDimension=2
  WheelRearRight : Concatenate  NumInputs=3  Mode=Multidimensional array  ConcatenateDimension=2
  ConcatOut : Outport  VectorParamsAs1DForOutWhenUnconnected=off
  wires:
  Body Yaw/1 -> Body/3
  WheelFrontLeft Yaw/1 -> WheelFrontLeft/3
  WheelFrontLeft/1 -> AllParts/2
  Body/1 -> AllParts/1
  WheelRearLeft/1 -> AllParts/4
  WheelFrontRight/1 -> AllParts/3
  WheelRearRight Yaw/1 -> WheelRearRight/3
  WheelRearLeft Yaw/1 -> WheelRearLeft/3
  AllParts/1 -> ConcatOut/1
  WheelRearRight/1 -> AllParts/5
  WheelFrontRight Yaw/1 -> WheelFrontRight/3
  Body Roll/1 -> Body/1
  Body Ptich/1 -> Body/2
  WheelFrontLeft Pitch/1 -> WheelFrontLeft/2
  WheelFrontLeft Roll/1 -> WheelFrontLeft/1
  WheelFrontRight Roll/1 -> WheelFrontRight/1
  WheelFrontRight Pitch/1 -> WheelFrontRight/2
  WheelRearLeft Roll/1 -> WheelRearLeft/1
  WheelRearLeft Pitch/1 -> WheelRearLeft/2
  WheelRearRight Roll/1 -> WheelRearRight/1
  WheelRearRight Ptich/1 -> WheelRearRight/2
